simulink model "lyskawaLab8_si"  (R2023b)
settings: Solver=VariableStepAuto  StartTime=startTime  StopTime=stopTime  MaxStep=maxStepSize  RelTol=1e-3
values from neighbouring files (symbols this model uses):
  dfwe1 = 0    [lyskawaLab8.m]
  dfwe2 = 0.1*fwe2max    [lyskawaLab8.m]
  h1_0 = fwe1_0/a1 + h2_0    [lyskawaLab8.m]
  h2_0 = (fwe1_0 + fwe2_0)/a2    [lyskawaLab8.m]
  L1 = [A2 a1+a2]    [lyskawaLab8.m]
  L2 = a1    [lyskawaLab8.m]
  L3 = a1    [lyskawaLab8.m]
  L4 = [A1 a1]    [lyskawaLab8.m]
  M = [A1*A2 A1*a1+A1*a2+A2*a1 a1*a2]    [lyskawaLab8.m]
  t0 = 5    [lyskawaLab8.m]
settings Model: Creator=aleklyskawa  LastModifiedBy=aleklyskawa

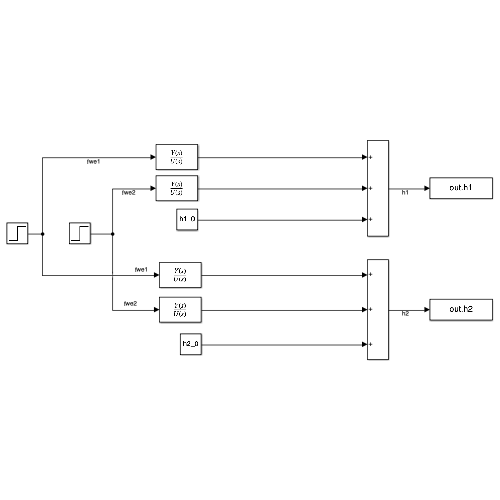
[thumbnail: Simulink's stored preview of the top-level diagram]
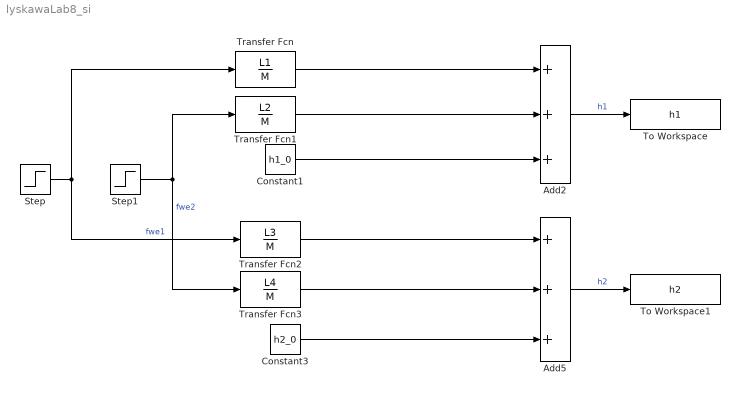
== system lyskawaLab8_si ==
  Add2 : Sum  Inputs=+++
  Add5 : Sum  Inputs=+++
  Constant1 : Constant  Value=h1_0
  Constant3 : Constant  Value=h2_0
  Step : Step  Time=t0  After=dfwe1  SampleTime=0
  Step1 : Step  Time=t0  After=dfwe2  SampleTime=0
  To Workspace : ToWorkspace  VariableName=h1  SampleTime=-1
  To Workspace1 : ToWorkspace  VariableName=h2  SampleTime=-1
  Transfer Fcn : TransferFcn  Numerator=L1  Denominator=M
  Transfer Fcn1 : TransferFcn  Numerator=L2  Denominator=M
  Transfer Fcn2 : TransferFcn  Numerator=L3  Denominator=M
  Transfer Fcn3 : TransferFcn  Numerator=L4  Denominator=M
  wires:
  Transfer Fcn/1 -> Add2/1
  Add5/1 -> To Workspace1/1  "h2"
  Transfer Fcn1/1 -> Add2/2
  Add2/1 -> To Workspace/1  "h1"
  Transfer Fcn2/1 -> Add5/1
  Step1/1 -> Transfer Fcn3/1, Transfer Fcn1/1  "fwe2"
  Constant3/1 -> Add5/3
  Transfer Fcn3/1 -> Add5/2
  Constant1/1 -> Add2/3
  Step/1 -> Transfer Fcn2/1, Transfer Fcn/1  "fwe1"
